simulink model "Subsystem"  (R2020b)
settings: Solver=VariableStepAuto  StartTime=0.0  StopTime=10.0  RelTol=1e-3
settings Model: Creator=MY lenovo  LastModifiedBy=MY lenovo
settings DataIOCC: SaveOutput=off  SaveTime=off

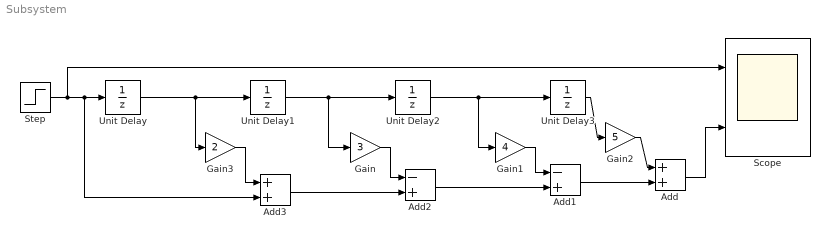
== system Subsystem ==
  Add : Sum
  Add1 : Sum  Inputs=-+
  Add2 : Sum  Inputs=-+
  Add3 : Sum
  Gain : Gain  Gain=3
  Gain1 : Gain  Gain=4
  Gain2 : Gain  Gain=5
  Gain3 : Gain  Gain=2
  Scope : Scope  NumInputPorts=2
  Step : Step  SampleTime=0
  Unit Delay{,1..3} (4 alike) : UnitDelay  SampleTime=-1  HasFrameUpgradeWarning=on
  wires:
  Add2/1 -> Add1/2
  Gain/1 -> Add2/1
  Unit Delay1/1 -> Unit Delay2/1, Gain/1
  Gain2/1 -> Add/1
  Add/1 -> Scope/2
  Unit Delay3/1 -> Gain2/1
  Gain3/1 -> Add3/1
  Step/1 -> Scope/1, Unit Delay/1, Add3/2
  Gain1/1 -> Add1/1
  Unit Delay2/1 -> Unit Delay3/1, Gain1/1
  Unit Delay/1 -> Unit Delay1/1, Gain3/1
  Add3/1 -> Add2/2
  Add1/1 -> Add/2
